simulink model "Exercise4_sim"  (R2020b)
settings: Solver=FixedStepAuto  StartTime=0.0  StopTime=1  FixedStep=Ts  RelTol=1e-5
undefined symbols (not defined in the file): C, L, R, ws
settings Model: Creator=mani8618  LastModifiedBy=kaidriscoll
settings DebuggingCC: SFMachineParentedDataDiag=error

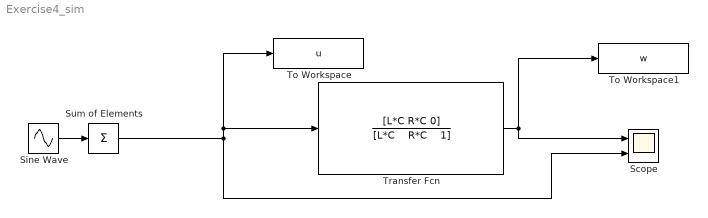
== system Exercise4_sim ==
  Scope : Scope  NumInputPorts=2
  Sine Wave : Sin  Frequency=ws  Phase=2*pi*rand(1,200)  SampleTime=0
  Sum of Elements : Sum  Inputs=+
  To Workspace : ToWorkspace  VariableName=u  SampleTime=-1
  To Workspace1 : ToWorkspace  VariableName=w  SampleTime=-1
  Transfer Fcn : TransferFcn  Numerator=[L*C R*C 0]  Denominator="[L*C    R*C    1]"
  wires:
  Transfer Fcn/1 -> Scope/1, To Workspace1/1
  Sine Wave/1 -> Sum of Elements/1
  Sum of Elements/1 -> To Workspace/1, Transfer Fcn/1, Scope/2
